simulink model "GSM"  (R2017b)
settings: Solver=VariableStepAuto  StartTime=0.0  StopTime=6  RelTol=1e-3
values from neighbouring files (symbols this model uses):
  cGSMP = block.DialogPrm(15).Data    [GSM_S.m]
  dcGSM = block.DialogPrm(9).Data    [GSM_S.m]
  dcP = block.DialogPrm(12).Data    [GSM_S.m]
  dGSMP = block.DialogPrm(16).Data    [GSM_S.m]
  dqP = block.DialogPrm(14).Data    [GSM_S.m]
  dvGSM = block.DialogPrm(10).Data    [GSM_S.m]
  dvP = block.DialogPrm(13).Data    [GSM_S.m]
  iGSM_0 = block.DialogPrm(1).Data    [GSM_S.m]
  JGSM = block.DialogPrm(8).Data    [GSM_S.m]
  JP = block.DialogPrm(11).Data    [GSM_S.m]
  kGSM = block.DialogPrm(7).Data    [GSM_S.m]
  LGSM = block.DialogPrm(5).Data    [GSM_S.m]
  phiGSMP_0 = block.DialogPrm(2).Data    [GSM_S.m]
  RGSM = block.DialogPrm(6).Data    [GSM_S.m]
  wGSM_0 = block.DialogPrm(3).Data    [GSM_S.m]
  wP_0 = block.DialogPrm(4).Data    [GSM_S.m]
undefined symbols (not defined in the file or in its folder): A, A_red, B, B_red, MextR, uGSMR
settings Model: Creator=user  LastModifiedBy=cristian-mac
settings SFSimCC: SimUseLocalCustomCode=on
settings RTWCC: RTWUseLocalCustomCode=on

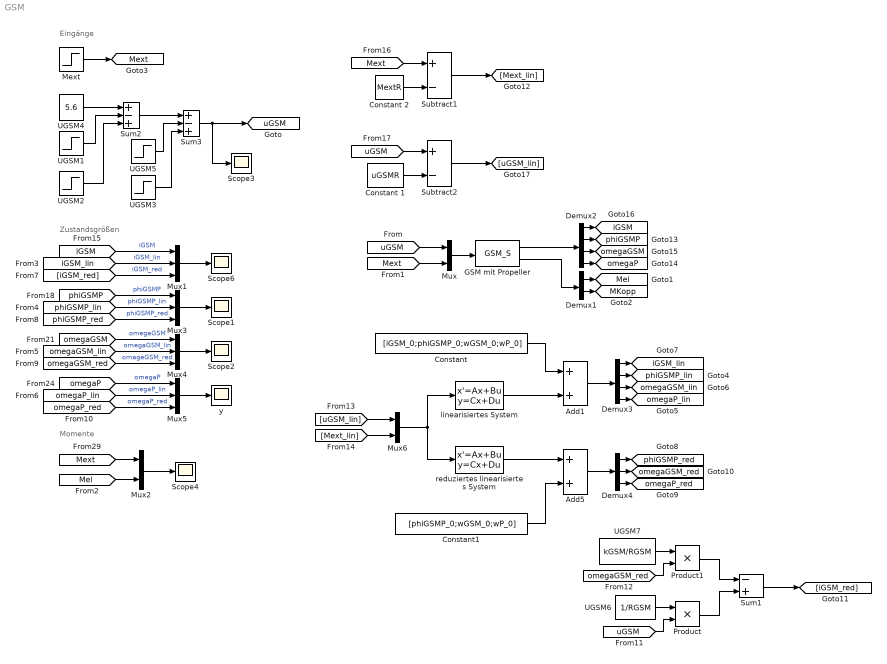
== system GSM ==
  note: Eingänge
  note: Momente
  note: Zustandsgrößen
  Add1 : Sum
  Add5 : Sum
  Constant : Constant  Value=[iGSM_0;phiGSMP_0;wGSM_0;wP_0]
  Constant 1 : Constant  Value=uGSMR
  Constant 2 : Constant  Value=MextR
  Constant1 : Constant  Value=[phiGSMP_0;wGSM_0;wP_0]
  Demux1 : Demux  Outputs=2
  Demux2 : Demux
  Demux3 : Demux
  Demux4 : Demux  Outputs=3
  GSM mit Propeller : M-S-Function  FunctionName=GSM_S  Parameters=iGSM_0, qGSMP_0, wGSM_0, wP_0, LGSM, RGSM, kGSM, JGSM, dcGSM, dvGSM, JP, dcP, dvP, dqP, cGSMP, dGSMP  mask{iGSM_0=iGSM_0, qGSMP_0=phiGSMP_0, wGSM_0=wGSM_0, wP_0=wP_0, LGSM=LGSM, RGSM=RGSM, kGSM=kGSM, JGSM=JGSM, dcGSM=dcGSM, dvGSM=dvGSM, JP=JP, dcP=dcP, dvP=dvP, dqP=dqP, cGSMP=cGSMP, dGSMP=dGSMP}
  Mext : Step  Time=11  After=0.25  SampleTime=0
  Mux : Mux  Inputs=2
  Mux{1,3..5} (4 alike) : Mux  Inputs=3
  Mux2 : Mux  Inputs=2
  Mux6 : Mux  Inputs=2
  Product : Product
  Product1 : Product
  Scope{1..4,6} (5 alike) : Scope
  Subtract1 : Sum  Inputs=+-
  Subtract2 : Sum  Inputs=+-
  Sum1 : Sum  Inputs=-+
  Sum2 : Sum  Inputs=+-+
  Sum3 : Sum  Inputs=+-+
  UGSM1 : Step  Time=2  SampleTime=0
  UGSM2 : Step  Time=5  SampleTime=0
  UGSM3 : Step  Time=13  After=2  SampleTime=0
  UGSM4 : Constant  Value=5.6
  UGSM5 : Step  Time=8  After=2  SampleTime=0
  UGSM6 : Constant  Value=1/RGSM
  UGSM7 : Constant  Value=kGSM/RGSM
  "linearisiertes System " : StateSpace  A=A  B=B  C=eye(4)  D=zeros(4,2)  InitialCondition=[0, 0, 0, 0]
  reduziertes linearisiertes System : StateSpace  A=A_red  B=B_red  C=eye(3)  D=zeros(3,2)  InitialCondition=[0, 0, 0]
  y : Scope
  tag scope: MKopp=global, Mel=global, Mext=global, iGSM=global, iGSM_lin=global, omegaGSM=global, omegaGSM_lin=global, omegaGSM_red=global, omegaP=global, omegaP_lin=global, omegaP_red=global, phiGSMP=global, phiGSMP_lin=global, phiGSMP_red=global, uGSM=global
  wires:
  [omegaP_red] -> Mux5/3  "omegaP_red"
  reduziertes linearisiertes System/1 -> Add5/1
  Constant1/1 -> Add5/2
  Demux3/2 -> [phiGSMP_lin]
  Sum2/1 -> Sum3/1
  Constant 1/1 -> Subtract2/2
  [omegaP] -> Mux5/1  "omegaP"
  Mux2/1 -> Scope4/1
  Demux4/1 -> [phiGSMP_red]
  [uGSM] -> Product/2
  UGSM6/1 -> Product/1
  UGSM7/1 -> Product1/1
  [uGSM_lin] -> Mux6/1
  Sum1/1 -> [iGSM_red]
  Add5/1 -> Demux4/1
  Product/1 -> Sum1/2
  Demux4/2 -> [omegaGSM_red]
  Product1/1 -> Sum1/1
  Subtract1/1 -> [Mext_lin]
  [iGSM_lin] -> Mux1/2  "iGSM_lin"
  Demux4/3 -> [omegaP_red]
  Mux6/1 -> "linearisiertes System "/1, reduziertes linearisiertes System/1
  Demux3/4 -> [omegaP_lin]
  [phiGSMP] -> Mux3/1  "phiGSMP"
  [omegaGSM_red] -> Mux4/3  "omageGSM_red"
  [omegaGSM_lin] -> Mux4/2  "omegaGSM_lin"
  [Mext_lin] -> Mux6/2
  [Mext] -> Mux/2
  Subtract2/1 -> [uGSM_lin]
  Mux5/1 -> y/1
  Mux3/1 -> Scope1/1
  [phiGSMP_lin] -> Mux3/2  "phiGSMP_lin"
  Constant/1 -> Add1/1
  Demux3/3 -> [omegaGSM_lin]
  [omegaGSM] -> Mux4/1  "omegaGSM"
  [uGSM] -> Mux/1
  Constant 2/1 -> Subtract1/2
  [iGSM] -> Mux1/1  "iGSM"
  UGSM4/1 -> Sum2/1
  [phiGSMP_red] -> Mux3/3  "phiGSMP_red"
  Demux1/1 -> [Mel]
  Demux2/3 -> [omegaGSM]
  Demux2/4 -> [omegaP]
  Demux1/2 -> [MKopp]
  UGSM3/1 -> Sum3/3
  Mux/1 -> GSM mit Propeller/1
  [iGSM_red] -> Mux1/3  "iGSM_red"
  [Mel] -> Mux2/2
  UGSM5/1 -> Sum3/2
  [Mext] -> Mux2/1
  Mux4/1 -> Scope2/1
  Demux2/2 -> [phiGSMP]
  Demux2/1 -> [iGSM]
  Add1/1 -> Demux3/1
  GSM mit Propeller/2 -> Demux1/1
  Demux3/1 -> [iGSM_lin]
  [Mext] -> Subtract1/1
  GSM mit Propeller/1 -> Demux2/1
  [omegaGSM_red] -> Product1/2
  UGSM1/1 -> Sum2/2
  [omegaP_lin] -> Mux5/2  "omegaP_lin"
  UGSM2/1 -> Sum2/3
  Mux1/1 -> Scope6/1
  [uGSM] -> Subtract2/1
  Mext/1 -> [Mext]
  Sum3/1 -> Scope3/1, [uGSM]
  "linearisiertes System "/1 -> Add1/2
